simulink library "Map"  (R2019b)
settings: Solver=VariableStepAuto  StartTime=0.0  StopTime=10.0  RelTol=1e-3
libraries: simulink x1
settings Model: Creator=Nick  LastModifiedBy=Nick
settings DataIOCC: ReturnWorkspaceOutputs=off
settings DebuggingCC: ArithmeticOperatorsInVariantConditions=warning
settings SFSimCC: CustomCodeUndefinedFunction=UseInterfaceOnly

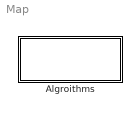
== system Map ==
  Algroithms : Subsystem

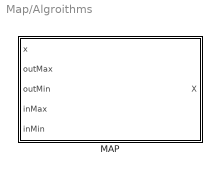
== system Map/Algroithms ==
  MAP : Subsystem

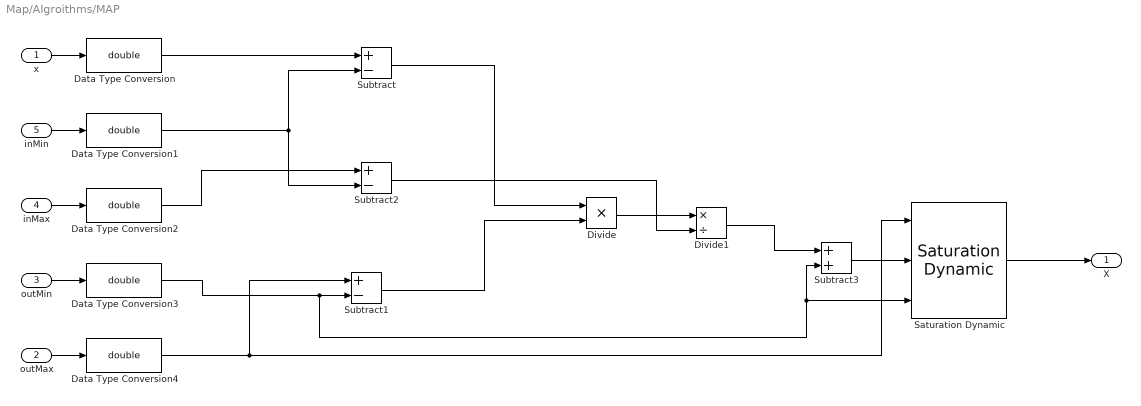
== system Map/Algroithms/MAP ==
  x : Inport
  outMax : Inport  Port=2
  outMin : Inport  Port=3
  inMax : Inport  Port=4
  inMin : Inport  Port=5
  Data Type Conversion{,1..4} (5 alike) : DataTypeConversion  OutDataTypeStr=double
  Divide : Product  Inputs=**
  Divide1 : Product  Inputs=*/
  Saturation Dynamic : simulink/Discontinuities/Saturation Dynamic  OutMin=[]  OutMax=[]  OutDataTypeStr=Inherit: Same as second input  OutDataType=fixdt(1, 16)  OutScaling=2^-10  DoSatur=off
  Subtract : Sum  Inputs=+-
  Subtract1 : Sum  Inputs=+-
  Subtract2 : Sum  Inputs=+-
  Subtract3 : Sum
  X : Outport
  wires:
  x/1 -> Data Type Conversion/1
  inMin/1 -> Data Type Conversion1/1
  Subtract/1 -> Divide/1
  outMax/1 -> Data Type Conversion4/1
  Data Type Conversion3/1 -> Saturation Dynamic/3, Subtract3/2, Subtract1/2
  Subtract1/1 -> Divide/2
  inMax/1 -> Data Type Conversion2/1
  Subtract2/1 -> Divide1/2
  Divide/1 -> Divide1/1
  Divide1/1 -> Subtract3/1
  Subtract3/1 -> Saturation Dynamic/2
  Saturation Dynamic/1 -> X/1
  Data Type Conversion/1 -> Subtract/1
  Data Type Conversion1/1 -> Subtract2/2, Subtract/2
  Data Type Conversion2/1 -> Subtract2/1
  outMin/1 -> Data Type Conversion3/1
  Data Type Conversion4/1 -> Saturation Dynamic/1, Subtract1/1
